simulink model "first"  (R2017a)
settings: Solver=VariableStepAuto  StartTime=0.0  StopTime=10.0  RelTol=1e-3
settings Model: Creator=Spars  LastModifiedBy=Spars

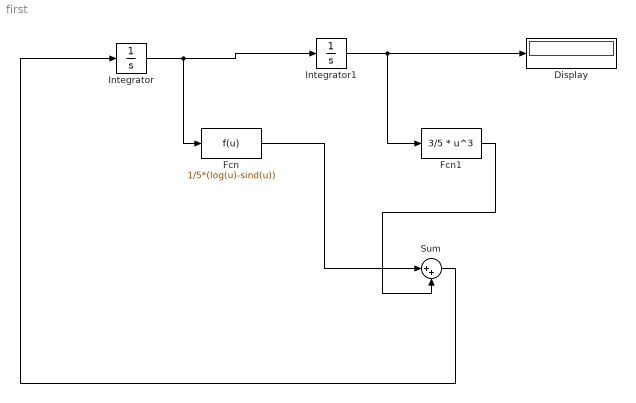
== system first ==
  Display : Display
  Fcn : Fcn  Expr=1/5*(log(u)-sind(u))
  Fcn1 : Fcn  Expr=3/5 * u^3
  Integrator : Integrator  LimitOutput=on  LowerSaturationLimit=0
  Integrator1 : Integrator
  Sum : Sum  Inputs=|++
  wires:
  Integrator/1 -> Fcn/1, Integrator1/1
  Integrator1/1 -> Display/1, Fcn1/1
  Fcn/1 -> Sum/1
  Fcn1/1 -> Sum/2
  Sum/1 -> Integrator/1
